simulink model "LQR_Control_block_project"  (R2018b)
settings: Solver=VariableStepAuto  StartTime=0.0  StopTime=160  RelTol=1e-3
values from neighbouring files (symbols this model uses):
  A = [0 1 0 0;-k1/m1 -b1/m1 k1/m1 b1/m1;0 0 0 1;k1/m2 b1/m2 (-k2-k1)/m2 -b1/m2]    [LQR_control_project.m]
  B = [0;1/m1;0; -1/m2 ]    [LQR_control_project.m]
  K = inv(R)*B'*P    [LQR_control_project.m]
settings Model: Creator=hp  LastModifiedBy=hp

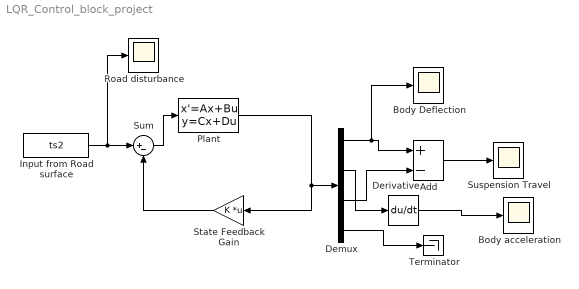
== system LQR_Control_block_project ==
  Add : Sum  Inputs=+-
  Body Deflection : Scope
      settings: Description=x_lablel=('time')
  Body acceleration : Scope
  Demux : Demux
  Derivative : Derivative
  Input from Road surface : FromWorkspace  VariableName=ts2  SampleTime=0
  "Plant " : StateSpace  A=A  B=B  C=eye(4)  D=[0;0;0;0]  InitialCondition=0
  Road disturbance : Scope
  State Feedback Gain : Gain  Gain=K  Multiplication=Matrix(K*u)  OutDataTypeStr=Inherit: Same as input
  Sum : Sum  Inputs=|+-
  Suspension Travel : Scope
  Terminator : Terminator
  wires:
  Input from Road surface/1 -> Road disturbance/1, Sum/1
  State Feedback Gain/1 -> Sum/2
  Sum/1 -> "Plant "/1
  "Plant "/1 -> State Feedback Gain/1, Demux/1
  Demux/1 -> Body Deflection/1, Add/1
  Demux/3 -> Add/2
  Add/1 -> Suspension Travel/1
  Demux/2 -> Derivative/1
  Derivative/1 -> Body acceleration/1
  Demux/4 -> Terminator/1
